simulink model "combined2"  (R2021a)
settings: Solver=VariableStepAuto  StartTime=0.0  StopTime=T_s  RelTol=1e-3
model workspace: external: MATLAB File C:\Users\abebe\Desktop\Matlab\solidworks\combined_DataFile.m (data not in the file)
values from neighbouring files (symbols this model uses):
  a_x = [0 0 0 0]    [starting_and_end_points.m]
  a_y = [10 40 30 10]    [starting_and_end_points.m]
  a_z = [30 30 30 30]    [starting_and_end_points.m]
  b_x = [0 0 0 0]    [starting_and_end_points.m]
  b_y = [40 30 10 3]    [starting_and_end_points.m]
  b_z = [30 30 30 30]    [starting_and_end_points.m]
  T = 2*max(A)    [starting_and_end_points.m]
  X = rf.*cos(PHI)    [meshing.m]
  Y = rf.*sin(PHI)    [meshing.m]
  Z = l1+(l2*sin(THETA1) + l3*sin(THETA1 + THETA2))    [meshing.m]
undefined symbols (not defined in the file or in its folder): smiData
libraries: sm_lib x20, nesl_utility x7, pid_lib x3
settings Model: Creator=Vogayer  LastModifiedBy=Vogayer

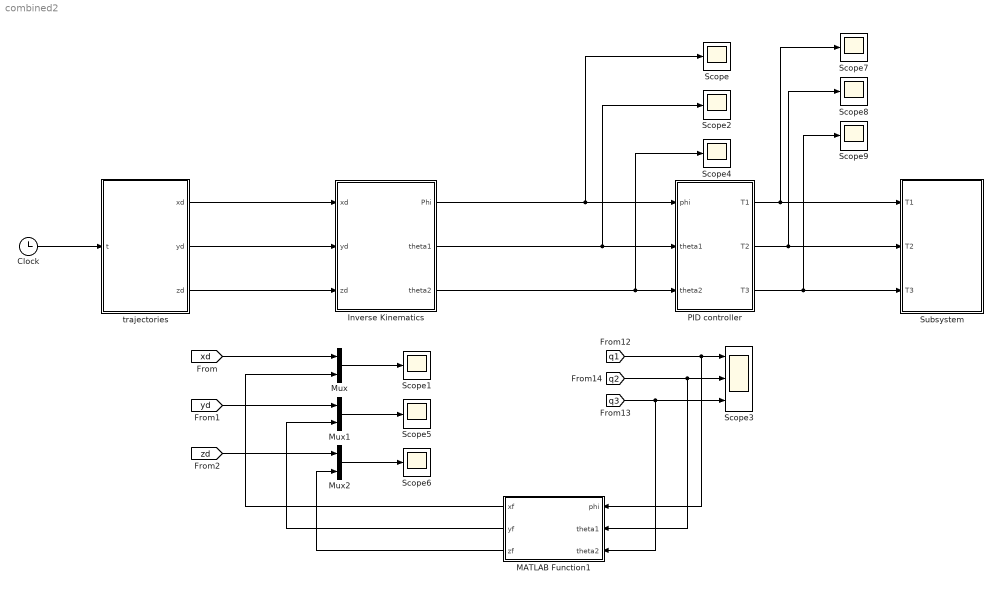
== system combined2 ==
  Clock : Clock
  Inverse Kinematics : Subsystem
  MATLAB Function1 : MATLAB Function  TreatAsAtomicUnit=on
  Mux : Mux  Inputs=2
  Mux1 : Mux  Inputs=2
  Mux2 : Mux  Inputs=2
  PID controller : Subsystem
  Scope{,1..2,4..9} (9 alike) : Scope
  Scope3 : Scope  NumInputPorts=3
  Subsystem : Subsystem
  trajectories : Subsystem
  wires:
  Inverse Kinematics/2(theta1) -> Scope2/1, PID controller/2(theta1)
  [xd] -> Mux/1
  MATLAB Function1/3(zf) -> Mux2/2
  Inverse Kinematics/3(theta2) -> Scope4/1, PID controller/3(theta2)
  MATLAB Function1/2(yf) -> Mux1/2
  [yd] -> Mux1/1
  Inverse Kinematics/1(Phi) -> Scope/1, PID controller/1(phi)
  [q2] -> MATLAB Function1/2(theta1), Scope3/2
  Mux2/1 -> Scope6/1
  [q3] -> MATLAB Function1/3(theta2), Scope3/3
  Mux/1 -> Scope1/1
  [zd] -> Mux2/1
  PID controller/1(T1) -> Subsystem/1(T1), Scope7/1
  Clock/1 -> trajectories/1(t)
  PID controller/2(T2) -> Subsystem/2(T2), Scope8/1
  Mux1/1 -> Scope5/1
  MATLAB Function1/1(xf) -> Mux/2
  [q1] -> MATLAB Function1/1(phi), Scope3/1
  PID controller/3(T3) -> Subsystem/3(T3), Scope9/1
  trajectories/1(xd) -> Inverse Kinematics/1(xd)
  trajectories/2(yd) -> Inverse Kinematics/2(yd)
  trajectories/3(zd) -> Inverse Kinematics/3(zd)

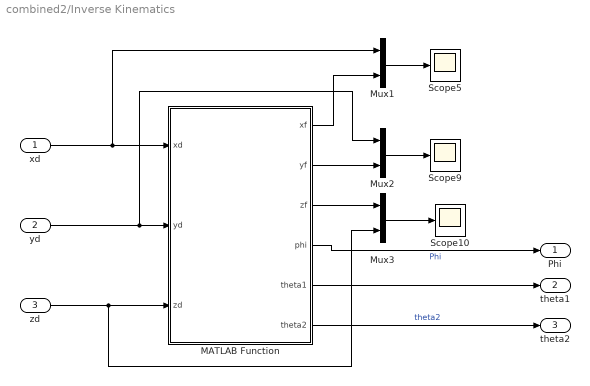
== system combined2/Inverse Kinematics ==
  xd : Inport
  yd : Inport  Port=2
  zd : Inport  Port=3
  MATLAB Function : MATLAB Function  TreatAsAtomicUnit=on
  Mux1 : Mux  Inputs=2
  Mux2 : Mux  Inputs=2
  Mux3 : Mux  Inputs=2
  Scope10 : Scope
  Scope5 : Scope
  Scope9 : Scope
  Phi : Outport
  theta1 : Outport  Port=2
  theta2 : Outport  Port=3
  wires:
  yd/1 -> MATLAB Function/2(yd), Mux2/1
  xd/1 -> MATLAB Function/1(xd), Mux1/1
  Mux2/1 -> Scope9/1
  MATLAB Function/3(zf) -> Mux3/1
  MATLAB Function/2(yf) -> Mux2/2
  Mux3/1 -> Scope10/1
  Mux1/1 -> Scope5/1
  zd/1 -> MATLAB Function/3(zd), Mux3/2
  MATLAB Function/1(xf) -> Mux1/2
  MATLAB Function/5(theta1) -> theta1/1
  MATLAB Function/4(phi) -> Phi/1  "Phi"
  MATLAB Function/6(theta2) -> theta2/1  "theta2"

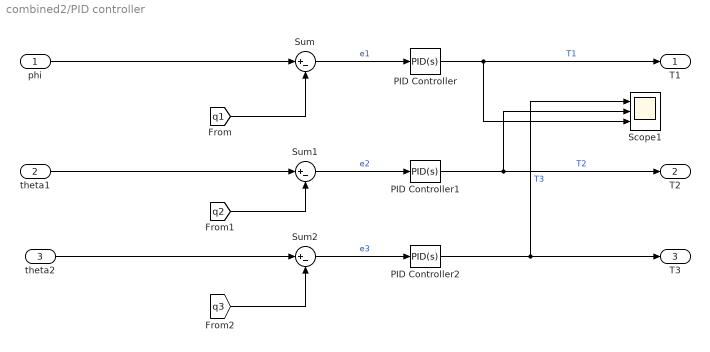
== system combined2/PID controller ==
  phi : Inport
  theta1 : Inport  Port=2
  theta2 : Inport  Port=3
  PID Controller : pid_lib/PID Controller  Controller=PID  Form=Parallel  TimeDomain=Continuous-time  UseExternalTs=off  SampleTime=-1  IntegratorMethod=Forward Euler  FilterMethod=Forward Euler  ControllerParametersSource=internal  P=2.28184982885174  I=1.06824293805434  D=1.19687109159291  UseFilter=on  N=54.5397025421619  TunerSelectOption=Transfer Function Based (PID Tuner App)  InitialConditionSource=internal  InitialConditionForIntegrator=0  InitialConditionForFilter=0  DifferentiatorICPrevScaledInput=0  ExternalReset=none  TrackingMode=off  Kt=1  LimitOutput=off  SatLimitsSource=internal  UpperSaturationLimit=inf  LowerSaturationLimit=-inf  LinearizeAsGain=on  AntiWindupMode=none  Kb=1  POutMin=[]  POutMax=[]  IOutMin=[]  IOutMax=[]  DOutMin=[]  DOutMax=[]  NOutMin=[]  NOutMax=[]  SumOutMin=[]  SumOutMax=[]  SaturationOutMin=[]  SaturationOutMax=[]  PParamMin=[]  PParamMax=[]  IParamMin=[]  IParamMax=[]  DParamMin=[]  DParamMax=[]  NParamMin=[]  NParamMax=[]  KbParamMin=[]  KbParamMax=[]  KtParamMin=[]  KtParamMax=[]  KbOutMin=[]  KbOutMax=[]  KtOutMin=[]  KtOutMax=[]  IntegratorOutMin=[]  IntegratorOutMax=[]  FilterOutMin=[]  FilterOutMax=[]  SumI1OutMin=[]  SumI1OutMax=[]  SumI2OutMin=[]  SumI2OutMax=[]  SumI3OutMin=[]  SumI3OutMax=[]  SumI4OutMin=[]  SumI4OutMax=[]  SumDOutMin=[]  SumDOutMax=[]  DifferentiatorOutMin=[]  DifferentiatorOutMax=[]  FilterDiffOutCoefMin=[]  FilterDiffOutCoefMax=[]  ReciprocalOutMin=[]  ReciprocalOutMax=[]  SumDenOutMin=[]  SumDenOutMax=[]  SumNumOutMin=[]  SumNumOutMax=[]  DivideOutMin=[]  DivideOutMax=[]  UdiffTsProdOutMin=[]  UdiffTsProdOutMax=[]  NTsProdOutMin=[]  NTsProdOutMax=[]  UintegralTsProdOutMin=[]  UintegralTsProdOutMax=[]  UngainTsProdOutMin=[]  UngainTsProdOutMax=[]  IntegratorContinuousStateAttributes=''  IntegratorStateMustResolveToSignalObject=off  IntegratorRTWStateStorageClass=Auto  FilterContinuousStateAttributes=''  FilterStateMustResolveToSignalObject=off  FilterRTWStateStorageClass=Auto  ParallelPVariant=InternalParameters  IdealPVariant=Disabled  IVariant=InternalParameters  DVariant=InternalParameters  IntegratorVariant=Continuous  SatVariant=Disabled  AWVariant=Passthrough  PCopyVariant=Disabled  TRVariant=Disabled  FdbkBlocksVariant=Forward  IdealPFdbkVariant=Disabled  SatFdbkVariant=Disabled  DerivativeFilterVariant=ContFilter  NVariant=InternalParameters  NCopyVariant=Disabled  FilterICVariant=InternalICsFilter  IntegratorICVariant=InternalICs  ExternalResetVariant=Disabled  TRSumVariant=Passthrough  SumFdbkVariant=Disabled  SumVariant=Sum_PID  TsampFilterVariant=InternalTs  TsampNgainVariant=Passthrough  TsampIntegralVariant=Passthrough  ExternalSaturationOutDataTypeStr=Inherit: Same as second input
  PID Controller1 : pid_lib/PID Controller  Controller=PID  Form=Parallel  TimeDomain=Continuous-time  UseExternalTs=off  SampleTime=-1  IntegratorMethod=Forward Euler  FilterMethod=Forward Euler  ControllerParametersSource=internal  P=66.3245976240351  I=108.858021997244  D=7.26461762494016  UseFilter=on  N=389.461376061763  TunerSelectOption=Transfer Function Based (PID Tuner App)  InitialConditionSource=internal  InitialConditionForIntegrator=0  InitialConditionForFilter=0  DifferentiatorICPrevScaledInput=0  ExternalReset=none  TrackingMode=off  Kt=1  LimitOutput=off  SatLimitsSource=internal  UpperSaturationLimit=inf  LowerSaturationLimit=-inf  LinearizeAsGain=on  AntiWindupMode=none  Kb=1  POutMin=[]  POutMax=[]  IOutMin=[]  IOutMax=[]  DOutMin=[]  DOutMax=[]  NOutMin=[]  NOutMax=[]  SumOutMin=[]  SumOutMax=[]  SaturationOutMin=[]  SaturationOutMax=[]  PParamMin=[]  PParamMax=[]  IParamMin=[]  IParamMax=[]  DParamMin=[]  DParamMax=[]  NParamMin=[]  NParamMax=[]  KbParamMin=[]  KbParamMax=[]  KtParamMin=[]  KtParamMax=[]  KbOutMin=[]  KbOutMax=[]  KtOutMin=[]  KtOutMax=[]  IntegratorOutMin=[]  IntegratorOutMax=[]  FilterOutMin=[]  FilterOutMax=[]  SumI1OutMin=[]  SumI1OutMax=[]  SumI2OutMin=[]  SumI2OutMax=[]  SumI3OutMin=[]  SumI3OutMax=[]  SumI4OutMin=[]  SumI4OutMax=[]  SumDOutMin=[]  SumDOutMax=[]  DifferentiatorOutMin=[]  DifferentiatorOutMax=[]  FilterDiffOutCoefMin=[]  FilterDiffOutCoefMax=[]  ReciprocalOutMin=[]  ReciprocalOutMax=[]  SumDenOutMin=[]  SumDenOutMax=[]  SumNumOutMin=[]  SumNumOutMax=[]  DivideOutMin=[]  DivideOutMax=[]  UdiffTsProdOutMin=[]  UdiffTsProdOutMax=[]  NTsProdOutMin=[]  NTsProdOutMax=[]  UintegralTsProdOutMin=[]  UintegralTsProdOutMax=[]  UngainTsProdOutMin=[]  UngainTsProdOutMax=[]  IntegratorContinuousStateAttributes=''  IntegratorStateMustResolveToSignalObject=off  IntegratorRTWStateStorageClass=Auto  FilterContinuousStateAttributes=''  FilterStateMustResolveToSignalObject=off  FilterRTWStateStorageClass=Auto  ParallelPVariant=InternalParameters  IdealPVariant=Disabled  IVariant=InternalParameters  DVariant=InternalParameters  IntegratorVariant=Continuous  SatVariant=Disabled  AWVariant=Passthrough  PCopyVariant=Disabled  TRVariant=Disabled  FdbkBlocksVariant=Forward  IdealPFdbkVariant=Disabled  SatFdbkVariant=Disabled  DerivativeFilterVariant=ContFilter  NVariant=InternalParameters  NCopyVariant=Disabled  FilterICVariant=InternalICsFilter  IntegratorICVariant=InternalICs  ExternalResetVariant=Disabled  TRSumVariant=Passthrough  SumFdbkVariant=Disabled  SumVariant=Sum_PID  TsampFilterVariant=InternalTs  TsampNgainVariant=Passthrough  TsampIntegralVariant=Passthrough  ExternalSaturationOutDataTypeStr=Inherit: Same as second input
  PID Controller2 : pid_lib/PID Controller  Controller=PID  Form=Parallel  TimeDomain=Continuous-time  UseExternalTs=off  SampleTime=-1  IntegratorMethod=Forward Euler  FilterMethod=Forward Euler  ControllerParametersSource=internal  P=92284.2323712411  I=28708337.0909785  D=65.6560213464691  UseFilter=on  N=51610.5658060228  TunerSelectOption=Transfer Function Based (PID Tuner App)  InitialConditionSource=internal  InitialConditionForIntegrator=0  InitialConditionForFilter=0  DifferentiatorICPrevScaledInput=0  ExternalReset=none  TrackingMode=off  Kt=1  LimitOutput=off  SatLimitsSource=internal  UpperSaturationLimit=inf  LowerSaturationLimit=-inf  LinearizeAsGain=on  AntiWindupMode=none  Kb=1  POutMin=[]  POutMax=[]  IOutMin=[]  IOutMax=[]  DOutMin=[]  DOutMax=[]  NOutMin=[]  NOutMax=[]  SumOutMin=[]  SumOutMax=[]  SaturationOutMin=[]  SaturationOutMax=[]  PParamMin=[]  PParamMax=[]  IParamMin=[]  IParamMax=[]  DParamMin=[]  DParamMax=[]  NParamMin=[]  NParamMax=[]  KbParamMin=[]  KbParamMax=[]  KtParamMin=[]  KtParamMax=[]  KbOutMin=[]  KbOutMax=[]  KtOutMin=[]  KtOutMax=[]  IntegratorOutMin=[]  IntegratorOutMax=[]  FilterOutMin=[]  FilterOutMax=[]  SumI1OutMin=[]  SumI1OutMax=[]  SumI2OutMin=[]  SumI2OutMax=[]  SumI3OutMin=[]  SumI3OutMax=[]  SumI4OutMin=[]  SumI4OutMax=[]  SumDOutMin=[]  SumDOutMax=[]  DifferentiatorOutMin=[]  DifferentiatorOutMax=[]  FilterDiffOutCoefMin=[]  FilterDiffOutCoefMax=[]  ReciprocalOutMin=[]  ReciprocalOutMax=[]  SumDenOutMin=[]  SumDenOutMax=[]  SumNumOutMin=[]  SumNumOutMax=[]  DivideOutMin=[]  DivideOutMax=[]  UdiffTsProdOutMin=[]  UdiffTsProdOutMax=[]  NTsProdOutMin=[]  NTsProdOutMax=[]  UintegralTsProdOutMin=[]  UintegralTsProdOutMax=[]  UngainTsProdOutMin=[]  UngainTsProdOutMax=[]  IntegratorContinuousStateAttributes=''  IntegratorStateMustResolveToSignalObject=off  IntegratorRTWStateStorageClass=Auto  FilterContinuousStateAttributes=''  FilterStateMustResolveToSignalObject=off  FilterRTWStateStorageClass=Auto  ParallelPVariant=InternalParameters  IdealPVariant=Disabled  IVariant=InternalParameters  DVariant=InternalParameters  IntegratorVariant=Continuous  SatVariant=Disabled  AWVariant=Passthrough  PCopyVariant=Disabled  TRVariant=Disabled  FdbkBlocksVariant=Forward  IdealPFdbkVariant=Disabled  SatFdbkVariant=Disabled  DerivativeFilterVariant=ContFilter  NVariant=InternalParameters  NCopyVariant=Disabled  FilterICVariant=InternalICsFilter  IntegratorICVariant=InternalICs  ExternalResetVariant=Disabled  TRSumVariant=Passthrough  SumFdbkVariant=Disabled  SumVariant=Sum_PID  TsampFilterVariant=InternalTs  TsampNgainVariant=Passthrough  TsampIntegralVariant=Passthrough  ExternalSaturationOutDataTypeStr=Inherit: Same as second input
  Scope1 : Scope  NumInputPorts=3
  Sum : Sum  Inputs=|+-
  Sum1 : Sum  Inputs=|+-
  Sum2 : Sum  Inputs=|+-
  T1 : Outport
  T2 : Outport  Port=2
  T3 : Outport  Port=3
  wires:
  Sum1/1 -> PID Controller1/1  "e2"
  Sum2/1 -> PID Controller2/1  "e3"
  theta2/1 -> Sum2/1
  [q3] -> Sum2/2
  [q1] -> Sum/2
  Sum/1 -> PID Controller/1  "e1"
  PID Controller2/1 -> Scope1/1, T3/1  "T3"
  phi/1 -> Sum/1
  theta1/1 -> Sum1/1
  PID Controller/1 -> T1/1, Scope1/3  "T1"
  [q2] -> Sum1/2
  PID Controller1/1 -> Scope1/2, T2/1  "T2"

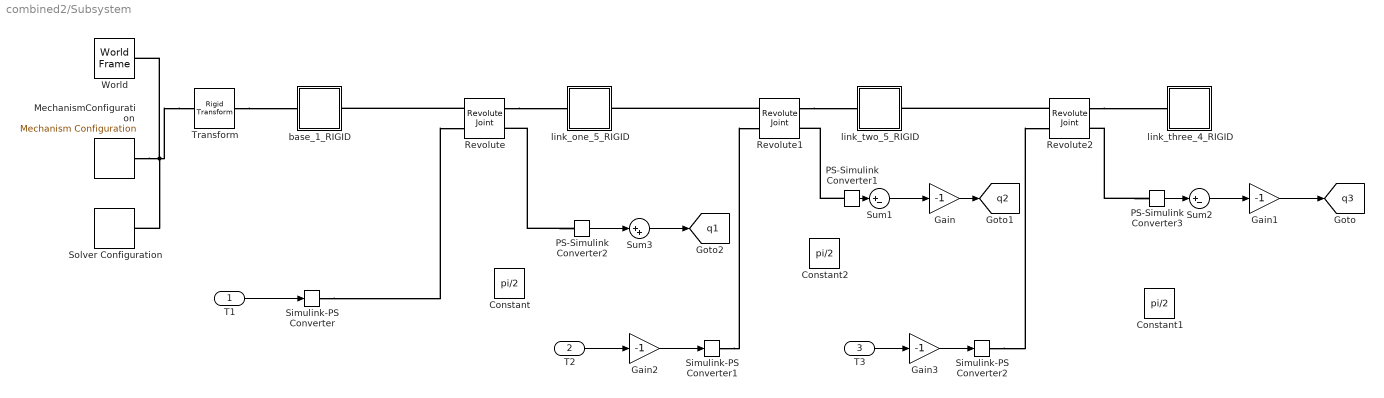
== system combined2/Subsystem ==
  T1 : Inport
  T2 : Inport  Port=2
  T3 : Inport  Port=3
  Constant : Constant  Value=pi/2
  Constant1 : Constant  Value=pi/2
  Constant2 : Constant  Value=pi/2
  Gain{,1..3} (4 alike) : Gain  Gain=-1
  MechanismConfiguration : sm_lib/Utilities/Mechanism Configuration  UniformGravity=Constant  GravityVector=[0 0 0]  GravityVectorUnits=m/s^2  GravityUnits=m/s^2  LinearizationDelta=0.001  JointModeTransitionNonlinearIterations=2
  PS-Simulink Converter1 : nesl_utility/PS-Simulink Converter  PhysicalDomain=network_engine_domain  SubClassName=ps_output  LeftPortType=input  RightPortType=output  PseudoPeriodic=off  Frequencies=[]  Unit=rad  AffineConversion=off
      settings: SourceProductBaseCode=PW,SS
  PS-Simulink Converter2 : nesl_utility/PS-Simulink Converter  PhysicalDomain=network_engine_domain  SubClassName=ps_output  LeftPortType=input  RightPortType=output  PseudoPeriodic=off  Frequencies=[]  Unit=rad  AffineConversion=off
      settings: SourceProductBaseCode=PW,SS
  PS-Simulink Converter3 : nesl_utility/PS-Simulink Converter  PhysicalDomain=network_engine_domain  SubClassName=ps_output  LeftPortType=input  RightPortType=output  PseudoPeriodic=off  Frequencies=[]  Unit=rad  AffineConversion=off
      settings: SourceProductBaseCode=PW,SS
  Revolute : sm_lib/Joints/Revolute Joint  JointMode=Normal  SenseConstraintForce=off  SenseConstraintForceX=off  SenseConstraintForceY=off  SenseConstraintForceZ=off  SenseConstraintTorque=off  SenseConstraintTorqueX=off  SenseConstraintTorqueY=off  SenseConstraintTorqueZ=off  SenseTotalForce=off  SenseTotalForceX=off  SenseTotalForceY=off  SenseTotalForceZ=off  SenseTotalTorque=off  SenseTotalTorqueX=off  SenseTotalTorqueY=off  SenseTotalTorqueZ=off  CompositeWrenchDir=FollowerOnBase  CompositeWrenchFrame=BaseFrame  EquilibriumPosition=0  EquilibriumPositionUnits=deg  SpringStiffness=0  SpringStiffnessUnits=N*m/deg  DampingCoefficient=0  DampingCoefficientUnits=N*m/(deg/s)  TorqueActuationMode=InputTorque  MotionActuationMode=ComputedMotion  SensePosition=on  SenseVelocity=off  SenseAcceleration=off  SenseTorqueForce=off  SenseLowerLimitTorqueForce=off  SenseUpperLimitTorqueForce=off  LowerLimitSpecify=off  LowerLimitBound=-90  LowerLimitBoundUnits=deg  LowerLimitStiffness=1e4  LowerLimitStiffnessUnits=N*m/deg  LowerLimitDamping=10  LowerLimitDampingUnits=N*m/(deg/s)  LowerLimitTransitionRegionWidth=0.1  LowerLimitTransitionRegionWidthUnits=deg  UpperLimitSpecify=off  UpperLimitBound=90  UpperLimitBoundUnits=deg  UpperLimitStiffness=1e4  UpperLimitStiffnessUnits=N*m/deg  UpperLimitDamping=10  UpperLimitDampingUnits=N*m/(deg/s)  UpperLimitTransitionRegionWidth=0.1  UpperLimitTransitionRegionWidthUnits=deg  PositionTargetSpecify=on  PositionTargetPriority=Low  PositionTargetValue=smiData.RevoluteJoint(1).Rz.Pos  PositionTargetValueUnits=deg  VelocityTargetSpecify=off  VelocityTargetPriority=High  VelocityTargetValue=0  VelocityTargetValueUnits=deg/s
  Revolute1 : sm_lib/Joints/Revolute Joint  JointMode=Normal  SenseConstraintForce=off  SenseConstraintForceX=off  SenseConstraintForceY=off  SenseConstraintForceZ=off  SenseConstraintTorque=off  SenseConstraintTorqueX=off  SenseConstraintTorqueY=off  SenseConstraintTorqueZ=off  SenseTotalForce=off  SenseTotalForceX=off  SenseTotalForceY=off  SenseTotalForceZ=off  SenseTotalTorque=off  SenseTotalTorqueX=off  SenseTotalTorqueY=off  SenseTotalTorqueZ=off  CompositeWrenchDir=FollowerOnBase  CompositeWrenchFrame=BaseFrame  EquilibriumPosition=0  EquilibriumPositionUnits=deg  SpringStiffness=0  SpringStiffnessUnits=N*m/deg  DampingCoefficient=0  DampingCoefficientUnits=N*m/(deg/s)  TorqueActuationMode=InputTorque  MotionActuationMode=ComputedMotion  SensePosition=on  SenseVelocity=off  SenseAcceleration=off  SenseTorqueForce=off  SenseLowerLimitTorqueForce=off  SenseUpperLimitTorqueForce=off  LowerLimitSpecify=off  LowerLimitBound=-90  LowerLimitBoundUnits=deg  LowerLimitStiffness=1e4  LowerLimitStiffnessUnits=N*m/deg  LowerLimitDamping=10  LowerLimitDampingUnits=N*m/(deg/s)  LowerLimitTransitionRegionWidth=0.1  LowerLimitTransitionRegionWidthUnits=deg  UpperLimitSpecify=off  UpperLimitBound=90  UpperLimitBoundUnits=deg  UpperLimitStiffness=1e4  UpperLimitStiffnessUnits=N*m/deg  UpperLimitDamping=10  UpperLimitDampingUnits=N*m/(deg/s)  UpperLimitTransitionRegionWidth=0.1  UpperLimitTransitionRegionWidthUnits=deg  PositionTargetSpecify=on  PositionTargetPriority=Low  PositionTargetValue=smiData.RevoluteJoint(2).Rz.Pos  PositionTargetValueUnits=deg  VelocityTargetSpecify=off  VelocityTargetPriority=High  VelocityTargetValue=0  VelocityTargetValueUnits=deg/s
  Revolute2 : sm_lib/Joints/Revolute Joint  JointMode=Normal  SenseConstraintForce=off  SenseConstraintForceX=off  SenseConstraintForceY=off  SenseConstraintForceZ=off  SenseConstraintTorque=off  SenseConstraintTorqueX=off  SenseConstraintTorqueY=off  SenseConstraintTorqueZ=off  SenseTotalForce=off  SenseTotalForceX=off  SenseTotalForceY=off  SenseTotalForceZ=off  SenseTotalTorque=off  SenseTotalTorqueX=off  SenseTotalTorqueY=off  SenseTotalTorqueZ=off  CompositeWrenchDir=FollowerOnBase  CompositeWrenchFrame=BaseFrame  EquilibriumPosition=0  EquilibriumPositionUnits=deg  SpringStiffness=0  SpringStiffnessUnits=N*m/deg  DampingCoefficient=0  DampingCoefficientUnits=N*m/(deg/s)  TorqueActuationMode=InputTorque  MotionActuationMode=ComputedMotion  SensePosition=on  SenseVelocity=off  SenseAcceleration=off  SenseTorqueForce=off  SenseLowerLimitTorqueForce=off  SenseUpperLimitTorqueForce=off  LowerLimitSpecify=off  LowerLimitBound=-90  LowerLimitBoundUnits=deg  LowerLimitStiffness=1e4  LowerLimitStiffnessUnits=N*m/deg  LowerLimitDamping=10  LowerLimitDampingUnits=N*m/(deg/s)  LowerLimitTransitionRegionWidth=0.1  LowerLimitTransitionRegionWidthUnits=deg  UpperLimitSpecify=off  UpperLimitBound=90  UpperLimitBoundUnits=deg  UpperLimitStiffness=1e4  UpperLimitStiffnessUnits=N*m/deg  UpperLimitDamping=10  UpperLimitDampingUnits=N*m/(deg/s)  UpperLimitTransitionRegionWidth=0.1  UpperLimitTransitionRegionWidthUnits=deg  PositionTargetSpecify=on  PositionTargetPriority=Low  PositionTargetValue=smiData.RevoluteJoint(3).Rz.Pos  PositionTargetValueUnits=deg  VelocityTargetSpecify=off  VelocityTargetPriority=High  VelocityTargetValue=0  VelocityTargetValueUnits=deg/s
  Simulink-PS Converter : nesl_utility/Simulink-PS Converter  PhysicalDomain=network_engine_domain  SubClassName=ps_input  LeftPortType=input  RightPortType=output  PseudoPeriodic=off  Frequencies=[]  NoiseDistribution=none  NoiseParameters=[]  Unit=N*m  AffineConversion=off  FilteringAndDerivatives=provide  SimscapeFilterOrder=1  InputFilterTimeConstant=0.001  UdotUserProvided=0
      settings: SourceProductBaseCode=PW,SS
  Simulink-PS Converter1 : nesl_utility/Simulink-PS Converter  PhysicalDomain=network_engine_domain  SubClassName=ps_input  LeftPortType=input  RightPortType=output  PseudoPeriodic=off  Frequencies=[]  NoiseDistribution=none  NoiseParameters=[]  Unit=N*m  AffineConversion=off  FilteringAndDerivatives=provide  SimscapeFilterOrder=1  InputFilterTimeConstant=0.001  UdotUserProvided=0
      settings: SourceProductBaseCode=PW,SS
  Simulink-PS Converter2 : nesl_utility/Simulink-PS Converter  PhysicalDomain=network_engine_domain  SubClassName=ps_input  LeftPortType=input  RightPortType=output  PseudoPeriodic=off  Frequencies=[]  NoiseDistribution=none  NoiseParameters=[]  Unit=N*m  AffineConversion=off  FilteringAndDerivatives=provide  SimscapeFilterOrder=1  InputFilterTimeConstant=0.001  UdotUserProvided=0
      settings: SourceProductBaseCode=PW,SS
  Solver Configuration : nesl_utility/Solver Configuration  PhysicalDomain=network_engine_domain  SubClassName=solver  LeftPortType=input  RightPortType=generic  Tones=[]  Harmonics=[]  SimulateNoise=off  Profile=off  UseLocalSampling=off  EnableSwitchedLinearOptims=on  FrequencyDomain=off  UseCCode=off  RelTol=0.001  AbsTol=1e-06  MinStep=1e-09  ToWorkspace=off  RevertToSquareIcSolve=off  NumHomotopyIterations=100  PhasorMode=off  PhasorModeNumHarmonics=1  DoDC=off  ResidualTolerance=1e-09  UseLocalSolver=off  LocalSolverChoice=NE_BACKWARD_EULER_ADVANCER  LocalSolverSampleTime=0.001  DoFixedCost=off  MaxNonlinIter=3  MaxModeIter=2  ComputeImpulses=off  ImpulseIterations=2  LinearAlgebra=auto  EquationFormulation=NE_TIME_EF  DelaysMemoryBudget=1024  AutomaticFiltering=on  FilteringTimeConstant=0.001  PartitionStorageMethod=AS_NEEDED  PartitionMemoryBudget=1024  PartitionMethod=ROBUST
      settings: SourceProductBaseCode=PW,SS
  Sum1 : Sum  Inputs=|+-
  Sum2 : Sum  Inputs=|+-
  Sum3 : Sum  Inputs=|++
  Transform : sm_lib/Frames and Transforms/Rigid Transform  TranslationMethod=Cartesian  TranslationStandardOffset=0  TranslationLengthUnit=cm  TranslationStandardAxis=+Z  TranslationCartesianOffset=smiData.RigidTransform(7).translation  TranslationROffset=0  TranslationROffsetUnits=m  TranslationZOffset=0  TranslationZOffsetUnits=m  TranslationThetaOffset=0  TranslationThetaOffsetUnits=deg  RotationMethod=ArbitraryAxis  RotationAngleUnits=rad  RotationStandardAxis=+Z  RotationAngle=smiData.RigidTransform(7).angle  RotationArbitraryAxis=smiData.RigidTransform(7).axis  FollAlignAxisA=+X  BaseAlignAxisA=+Y  FollAlignAxisB=+Y  BaseAlignAxisB=+Z  RotationSequenceAxes=FollowerAxes  RotationSequence=XYX  RotationSequenceAngles=[0 0 0]  RotationSequenceAnglesUnits=deg  RotationMatrix=[1 0 0; 0 1 0; 0 0 1]
  World : sm_lib/Frames and Transforms/World Frame
  base_1_RIGID : Subsystem
  link_one_5_RIGID : Subsystem
  link_three_4_RIGID : Subsystem
  link_two_5_RIGID : Subsystem
  tag scope: q1=global, q2=global, q3=global
  wires:
  T1/1 -> Simulink-PS Converter/1
  T3/1 -> Gain3/1
  T2/1 -> Gain2/1
  Sum3/1 -> [q1]
  Sum1/1 -> Gain/1
  PS-Simulink Converter1/1 -> Sum1/1
  PS-Simulink Converter3/1 -> Sum2/1
  PS-Simulink Converter2/1 -> Sum3/1
  Gain/1 -> [q2]
  Sum2/1 -> Gain1/1
  Gain1/1 -> [q3]
  Gain2/1 -> Simulink-PS Converter1/1
  Gain3/1 -> Simulink-PS Converter2/1
  connections:
  PS-Simulink Converter3/LConn1 -- Revolute2/RConn2
  Transform/LConn1 -- MechanismConfiguration/RConn1 -- Solver Configuration/RConn1 -- World/RConn1
  Simulink-PS Converter/RConn1 -- Revolute/LConn2
  Simulink-PS Converter2/RConn1 -- Revolute2/LConn2
  PS-Simulink Converter2/LConn1 -- Revolute/RConn2
  Revolute1/LConn1 -- link_one_5_RIGID/RConn1
  Transform/RConn1 -- base_1_RIGID/LConn1
  Revolute2/RConn1 -- link_three_4_RIGID/LConn1
  Revolute/RConn1 -- link_one_5_RIGID/LConn1
  Simulink-PS Converter1/RConn1 -- Revolute1/LConn2
  Revolute/LConn1 -- base_1_RIGID/RConn1
  PS-Simulink Converter1/LConn1 -- Revolute1/RConn2
  Revolute2/LConn1 -- link_two_5_RIGID/RConn1
  Revolute1/RConn1 -- link_two_5_RIGID/LConn1

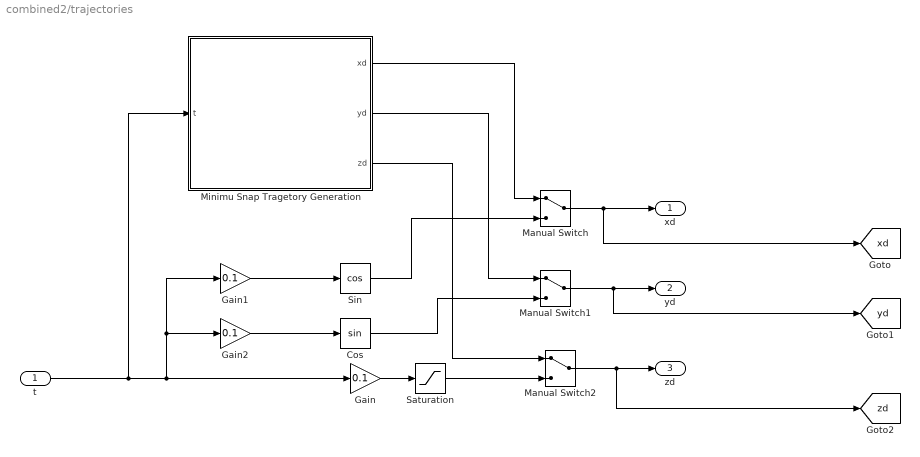
== system combined2/trajectories ==
  t : Inport
  Cos : Trigonometry
  Gain : Gain  Gain=0.1
  Gain1 : Gain  Gain=0.1
  Gain2 : Gain  Gain=0.1
  Manual Switch : ManualSwitch
  Manual Switch1 : ManualSwitch
  Manual Switch2 : ManualSwitch
  Minimu Snap Tragetory Generation : Subsystem
  Saturation : Saturate  LowerLimit=0
  Sin : Trigonometry  Operator=cos
  xd : Outport
  yd : Outport  Port=2
  zd : Outport  Port=3
  tag scope: xd=global, yd=global, zd=global
  wires:
  Cos/1 -> Manual Switch1/2
  Gain/1 -> Saturation/1
  t/1 -> Minimu Snap Tragetory Generation/1(t), Gain1/1, Gain2/1, Gain/1
  Minimu Snap Tragetory Generation/3(zd) -> Manual Switch2/1
  Minimu Snap Tragetory Generation/1(xd) -> Manual Switch/1
  Minimu Snap Tragetory Generation/2(yd) -> Manual Switch1/1
  Gain1/1 -> Sin/1
  Sin/1 -> Manual Switch/2
  Gain2/1 -> Cos/1
  Manual Switch/1 -> [xd], xd/1
  Manual Switch2/1 -> [zd], zd/1
  Manual Switch1/1 -> [yd], yd/1
  Saturation/1 -> Manual Switch2/2

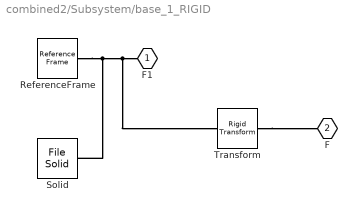
== system combined2/Subsystem/base_1_RIGID ==
  ReferenceFrame : sm_lib/Frames and Transforms/Reference Frame
  Solid : sm_lib/Body Elements/File Solid  ExtGeomFileName=base_Default_sldprt.STEP  UnitType=FromFile  ExtGeomFileUnits=m  StepReaderType=HEX  ExportConvexHullGeometry=off  InertiaType=Custom  Mass=smiData.Solid(4).mass  MassUnits=kg  CenterOfMass=smiData.Solid(4).CoM  CenterOfMassUnits=cm  MomentsOfInertia=smiData.Solid(4).MoI  MomentsOfInertiaUnits=kg*cm^2  ProductsOfInertia=smiData.Solid(4).PoI  ProductsOfInertiaUnits=kg*cm^2  BasedOnType=DensityFromFile  Density=1000  DensityUnits=kg/m^3  DoExposeReferenceFrame=on  SerializedFrames=<Frames/>  GraphicType=FromGeometry  MarkerShape=Sphere  MarkerSize=10  GraphicVisPropType=SimpleVisualProperties  GraphicDiffuseColor=smiData.Solid(4).color  GraphicSpecularColor=[0.5 0.5 0.5 1.0]  GraphicAmbientColor=[0.15 0.15 0.15 1.0]  GraphicEmissiveColor=[0.0 0.0 0.0 1.0]  GraphicShininess=75  GraphicOpacity=smiData.Solid(4).opacity
  Transform : sm_lib/Frames and Transforms/Rigid Transform  TranslationMethod=Cartesian  TranslationStandardOffset=0  TranslationLengthUnit=cm  TranslationStandardAxis=+Z  TranslationCartesianOffset=smiData.RigidTransform(1).translation  TranslationROffset=0  TranslationROffsetUnits=m  TranslationZOffset=0  TranslationZOffsetUnits=m  TranslationThetaOffset=0  TranslationThetaOffsetUnits=deg  RotationMethod=ArbitraryAxis  RotationAngleUnits=rad  RotationStandardAxis=+Z  RotationAngle=smiData.RigidTransform(1).angle  RotationArbitraryAxis=smiData.RigidTransform(1).axis  FollAlignAxisA=+X  BaseAlignAxisA=+Y  FollAlignAxisB=+Y  BaseAlignAxisB=+Z  RotationSequenceAxes=FollowerAxes  RotationSequence=XYX  RotationSequenceAngles=[0 0 0]  RotationSequenceAnglesUnits=deg  RotationMatrix=[1 0 0; 0 1 0; 0 0 1]
  F1 : PMIOPort  Side=Left
  F : PMIOPort  Port=2  Side=Right
  connections:
  Solid/RConn1 -- ReferenceFrame/RConn1 -- Transform/LConn1 -- F1/RConn1
  Transform/RConn1 -- F/RConn1

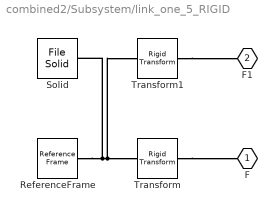
== system combined2/Subsystem/link_one_5_RIGID ==
  ReferenceFrame : sm_lib/Frames and Transforms/Reference Frame
  Solid : sm_lib/Body Elements/File Solid  ExtGeomFileName=link one_Default_sldprt.STEP  UnitType=FromFile  ExtGeomFileUnits=m  StepReaderType=HEX  ExportConvexHullGeometry=off  InertiaType=Custom  Mass=smiData.Solid(1).mass  MassUnits=kg  CenterOfMass=smiData.Solid(1).CoM  CenterOfMassUnits=cm  MomentsOfInertia=smiData.Solid(1).MoI  MomentsOfInertiaUnits=kg*cm^2  ProductsOfInertia=smiData.Solid(1).PoI  ProductsOfInertiaUnits=kg*cm^2  BasedOnType=DensityFromFile  Density=1000  DensityUnits=kg/m^3  DoExposeReferenceFrame=on  SerializedFrames=<Frames/>  GraphicType=FromGeometry  MarkerShape=Sphere  MarkerSize=10  GraphicVisPropType=SimpleVisualProperties  GraphicDiffuseColor=smiData.Solid(1).color  GraphicSpecularColor=[0.5 0.5 0.5 1.0]  GraphicAmbientColor=[0.15 0.15 0.15 1.0]  GraphicEmissiveColor=[0.0 0.0 0.0 1.0]  GraphicShininess=75  GraphicOpacity=smiData.Solid(1).opacity
  Transform : sm_lib/Frames and Transforms/Rigid Transform  TranslationMethod=Cartesian  TranslationStandardOffset=0  TranslationLengthUnit=cm  TranslationStandardAxis=+Z  TranslationCartesianOffset=smiData.RigidTransform(2).translation  TranslationROffset=0  TranslationROffsetUnits=m  TranslationZOffset=0  TranslationZOffsetUnits=m  TranslationThetaOffset=0  TranslationThetaOffsetUnits=deg  RotationMethod=ArbitraryAxis  RotationAngleUnits=rad  RotationStandardAxis=+Z  RotationAngle=smiData.RigidTransform(2).angle  RotationArbitraryAxis=smiData.RigidTransform(2).axis  FollAlignAxisA=+X  BaseAlignAxisA=+Y  FollAlignAxisB=+Y  BaseAlignAxisB=+Z  RotationSequenceAxes=FollowerAxes  RotationSequence=XYX  RotationSequenceAngles=[0 0 0]  RotationSequenceAnglesUnits=deg  RotationMatrix=[1 0 0; 0 1 0; 0 0 1]
  Transform1 : sm_lib/Frames and Transforms/Rigid Transform  TranslationMethod=Cartesian  TranslationStandardOffset=0  TranslationLengthUnit=cm  TranslationStandardAxis=+Z  TranslationCartesianOffset=smiData.RigidTransform(3).translation  TranslationROffset=0  TranslationROffsetUnits=m  TranslationZOffset=0  TranslationZOffsetUnits=m  TranslationThetaOffset=0  TranslationThetaOffsetUnits=deg  RotationMethod=ArbitraryAxis  RotationAngleUnits=rad  RotationStandardAxis=+Z  RotationAngle=smiData.RigidTransform(3).angle  RotationArbitraryAxis=smiData.RigidTransform(3).axis  FollAlignAxisA=+X  BaseAlignAxisA=+Y  FollAlignAxisB=+Y  BaseAlignAxisB=+Z  RotationSequenceAxes=FollowerAxes  RotationSequence=XYX  RotationSequenceAngles=[0 0 0]  RotationSequenceAnglesUnits=deg  RotationMatrix=[1 0 0; 0 1 0; 0 0 1]
  F : PMIOPort  Side=Left
  F1 : PMIOPort  Port=2  Side=Right
  connections:
  Solid/RConn1 -- ReferenceFrame/RConn1 -- Transform/LConn1 -- Transform1/LConn1
  Transform/RConn1 -- F/RConn1
  Transform1/RConn1 -- F1/RConn1

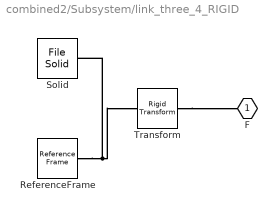
== system combined2/Subsystem/link_three_4_RIGID ==
  ReferenceFrame : sm_lib/Frames and Transforms/Reference Frame
  Solid : sm_lib/Body Elements/File Solid  ExtGeomFileName=link three_Default_sldprt.STEP  UnitType=FromFile  ExtGeomFileUnits=m  StepReaderType=HEX  ExportConvexHullGeometry=off  InertiaType=Custom  Mass=smiData.Solid(2).mass  MassUnits=kg  CenterOfMass=smiData.Solid(2).CoM  CenterOfMassUnits=cm  MomentsOfInertia=smiData.Solid(2).MoI  MomentsOfInertiaUnits=kg*cm^2  ProductsOfInertia=smiData.Solid(2).PoI  ProductsOfInertiaUnits=kg*cm^2  BasedOnType=DensityFromFile  Density=1000  DensityUnits=kg/m^3  DoExposeReferenceFrame=on  SerializedFrames=<Frames/>  GraphicType=FromGeometry  MarkerShape=Sphere  MarkerSize=10  GraphicVisPropType=SimpleVisualProperties  GraphicDiffuseColor=smiData.Solid(2).color  GraphicSpecularColor=[0.5 0.5 0.5 1.0]  GraphicAmbientColor=[0.15 0.15 0.15 1.0]  GraphicEmissiveColor=[0.0 0.0 0.0 1.0]  GraphicShininess=75  GraphicOpacity=smiData.Solid(2).opacity
  Transform : sm_lib/Frames and Transforms/Rigid Transform  TranslationMethod=Cartesian  TranslationStandardOffset=0  TranslationLengthUnit=cm  TranslationStandardAxis=+Z  TranslationCartesianOffset=smiData.RigidTransform(6).translation  TranslationROffset=0  TranslationROffsetUnits=m  TranslationZOffset=0  TranslationZOffsetUnits=m  TranslationThetaOffset=0  TranslationThetaOffsetUnits=deg  RotationMethod=ArbitraryAxis  RotationAngleUnits=rad  RotationStandardAxis=+Z  RotationAngle=smiData.RigidTransform(6).angle  RotationArbitraryAxis=smiData.RigidTransform(6).axis  FollAlignAxisA=+X  BaseAlignAxisA=+Y  FollAlignAxisB=+Y  BaseAlignAxisB=+Z  RotationSequenceAxes=FollowerAxes  RotationSequence=XYX  RotationSequenceAngles=[0 0 0]  RotationSequenceAnglesUnits=deg  RotationMatrix=[1 0 0; 0 1 0; 0 0 1]
  F : PMIOPort  Side=Left
  connections:
  Solid/RConn1 -- ReferenceFrame/RConn1 -- Transform/LConn1
  Transform/RConn1 -- F/RConn1

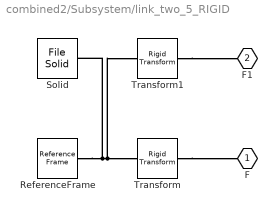
== system combined2/Subsystem/link_two_5_RIGID ==
  ReferenceFrame : sm_lib/Frames and Transforms/Reference Frame
  Solid : sm_lib/Body Elements/File Solid  ExtGeomFileName=link two_Default_sldprt.STEP  UnitType=FromFile  ExtGeomFileUnits=m  StepReaderType=HEX  ExportConvexHullGeometry=off  InertiaType=Custom  Mass=smiData.Solid(3).mass  MassUnits=kg  CenterOfMass=smiData.Solid(3).CoM  CenterOfMassUnits=cm  MomentsOfInertia=smiData.Solid(3).MoI  MomentsOfInertiaUnits=kg*cm^2  ProductsOfInertia=smiData.Solid(3).PoI  ProductsOfInertiaUnits=kg*cm^2  BasedOnType=DensityFromFile  Density=1000  DensityUnits=kg/m^3  DoExposeReferenceFrame=on  SerializedFrames=<Frames/>  GraphicType=FromGeometry  MarkerShape=Sphere  MarkerSize=10  GraphicVisPropType=SimpleVisualProperties  GraphicDiffuseColor=smiData.Solid(3).color  GraphicSpecularColor=[0.5 0.5 0.5 1.0]  GraphicAmbientColor=[0.15 0.15 0.15 1.0]  GraphicEmissiveColor=[0.0 0.0 0.0 1.0]  GraphicShininess=75  GraphicOpacity=smiData.Solid(3).opacity
  Transform : sm_lib/Frames and Transforms/Rigid Transform  TranslationMethod=Cartesian  TranslationStandardOffset=0  TranslationLengthUnit=cm  TranslationStandardAxis=+Z  TranslationCartesianOffset=smiData.RigidTransform(4).translation  TranslationROffset=0  TranslationROffsetUnits=m  TranslationZOffset=0  TranslationZOffsetUnits=m  TranslationThetaOffset=0  TranslationThetaOffsetUnits=deg  RotationMethod=ArbitraryAxis  RotationAngleUnits=rad  RotationStandardAxis=+Z  RotationAngle=smiData.RigidTransform(4).angle  RotationArbitraryAxis=smiData.RigidTransform(4).axis  FollAlignAxisA=+X  BaseAlignAxisA=+Y  FollAlignAxisB=+Y  BaseAlignAxisB=+Z  RotationSequenceAxes=FollowerAxes  RotationSequence=XYX  RotationSequenceAngles=[0 0 0]  RotationSequenceAnglesUnits=deg  RotationMatrix=[1 0 0; 0 1 0; 0 0 1]
  Transform1 : sm_lib/Frames and Transforms/Rigid Transform  TranslationMethod=Cartesian  TranslationStandardOffset=0  TranslationLengthUnit=cm  TranslationStandardAxis=+Z  TranslationCartesianOffset=smiData.RigidTransform(5).translation  TranslationROffset=0  TranslationROffsetUnits=m  TranslationZOffset=0  TranslationZOffsetUnits=m  TranslationThetaOffset=0  TranslationThetaOffsetUnits=deg  RotationMethod=ArbitraryAxis  RotationAngleUnits=rad  RotationStandardAxis=+Z  RotationAngle=smiData.RigidTransform(5).angle  RotationArbitraryAxis=smiData.RigidTransform(5).axis  FollAlignAxisA=+X  BaseAlignAxisA=+Y  FollAlignAxisB=+Y  BaseAlignAxisB=+Z  RotationSequenceAxes=FollowerAxes  RotationSequence=XYX  RotationSequenceAngles=[0 0 0]  RotationSequenceAnglesUnits=deg  RotationMatrix=[1 0 0; 0 1 0; 0 0 1]
  F : PMIOPort  Side=Left
  F1 : PMIOPort  Port=2  Side=Right
  connections:
  Solid/RConn1 -- ReferenceFrame/RConn1 -- Transform/LConn1 -- Transform1/LConn1
  Transform/RConn1 -- F/RConn1
  Transform1/RConn1 -- F1/RConn1

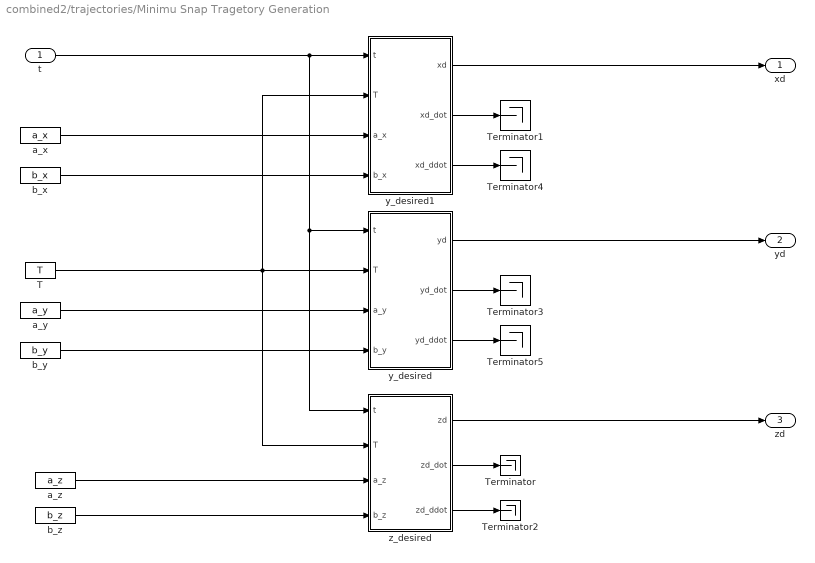
== system combined2/trajectories/Minimu Snap Tragetory Generation ==
  t : Inport
  " z_desired" : MATLAB Function  TreatAsAtomicUnit=on
  T : Constant  Value=T
  Terminator{,1..5} (6 alike) : Terminator
  a_x : Constant  Value=a_x
  a_y : Constant  Value=a_y
  a_z : Constant  Value=a_z
  b_x : Constant  Value=b_x
  b_y : Constant  Value=b_y
  b_z : Constant  Value=b_z
  y_desired : MATLAB Function  TreatAsAtomicUnit=on
  y_desired1 : MATLAB Function  TreatAsAtomicUnit=on
  xd : Outport
  yd : Outport  Port=2
  zd : Outport  Port=3
  wires:
  " z_desired"/3(zd_ddot) -> Terminator2/1
  " z_desired"/2(zd_dot) -> Terminator/1
  t/1 -> y_desired1/1(t), " z_desired"/1(t), y_desired/1(t)
  y_desired/2(yd_dot) -> Terminator3/1
  a_z/1 -> " z_desired"/3(a_z)
  T/1 -> y_desired1/2(T), " z_desired"/2(T), y_desired/2(T)
  y_desired1/1(xd) -> xd/1
  y_desired/1(yd) -> yd/1
  a_y/1 -> y_desired/3(a_y)
  b_z/1 -> " z_desired"/4(b_z)
  y_desired1/2(xd_dot) -> Terminator1/1
  " z_desired"/1(zd) -> zd/1
  b_y/1 -> y_desired/4(b_y)
  y_desired/3(yd_ddot) -> Terminator5/1
  y_desired1/3(xd_ddot) -> Terminator4/1
  a_x/1 -> y_desired1/3(a_x)
  b_x/1 -> y_desired1/4(b_x)

== matlab function combined2/Inverse Kinematics/MATLAB Function ==
  data: xd input; xf output; yd input; zd input; yf output; zf output; phi output; theta1 output; theta2 output
function [xf,yf,zf,phi,theta1,theta2] = fcn(xd,yd,zd)
l1=28;l2=40;l3=40;
phi=atan2(yd,xd);
r=sqrt(xd^2 + yd^2);
c2 = (r^2 + (zd-l1)^2 - l2^2 - l3^2)/(2*l2*l3);
s2=sqrt(1 - c2^2);
theta2=-atan2(s2,c2);
beta=-atan((l3*sin(theta2))/(l2 + l3*cos(theta2)));
gama=atan((zd-l1)/r);
theta1=gama-beta;
rf=l2*cos(theta1) + l3*cos((theta1-theta2));
zf=l1+(l2*sin(theta1) + l3*sin(theta1-theta2));
xf=rf*cos(phi);
yf=rf*sin(phi);

== matlab function combined2/MATLAB Function1 ==
  data: phi input; xf output; theta1 input; theta2 input; yf output; zf output
function [xf,yf,zf] = fcn(phi,theta1,theta2)
l1=28;l2=40;l3=40;
rf=l2*cos(theta1) + l3*cos((theta1-theta2));
zf=l1+(l2*sin(theta1) + l3*sin(theta1-theta2));
xf=rf*cos(phi);
yf=rf*sin(phi);

== matlab function combined2/trajectories/Minimu Snap Tragetory Generation/y_desired1 ==
  data: t input; T input; xd output; xd_dot output; xd_ddot output; a_x input; b_x input
function [xd,xd_dot,xd_ddot] = fcn(t,T,a_x,b_x)
if(t<=T(1,1))
T0=0;Tf=T(1,1);
a=a_x(1,1); b=b_x(1,1);
elseif(t>T(1,1)&& t<=T(2,1)+T(1,1))
T0=T(1,1);Tf=T(2,1)+T(1,1);
a=a_x(2,1); b=b_x(2,1);
elseif (t>T(2,1)+T(1,1)&& t<=T(3,1) + T(2,1)+T(1,1))
T0=T(2,1)+T(1,1);Tf=T(3,1)+ T(2,1)+T(1,1);
a=a_x(3,1); b=b_x(3,1);
else
T0=T(3,1)+ T(2,1)+T(1,1);Tf=T(4,1) + T(3,1)+ T(2,1)+T(1,1);
a=a_x(4,1); b=b_x(4,1);
end
B=[a;b;0;0;0;0;0;0];
A=[T0^6     T0^5     T0^4     T0^3    T0^2  T0^1  1;
   Tf^6     Tf^5     Tf^4     Tf^3    Tf^2  Tf^1  1;
   6*T0^5   5*T0^4   4*T0^3   3*T0^2  2*T0  1     0;
   6*Tf^5   5*Tf^4   4*Tf^3   3*Tf^2  2*Tf  1     0;
   30*T0^4  20*T0^3  12*T0^2  6*T0    2     0     0;
   30*Tf^4  20*Tf^3  12*Tf^2  6*Tf    2     0     0;
   120*T0^3  60*T0^2  24*T0   6       2     0     0;
   120*Tf^3  60*Tf^2  24*Tf   6       2     0     0];
C=A\B;
xd=C(1,1)*t^6 + C(2,1)*t^5 + C(3,1)*t^4 + C(4,1)*t^3 + C(5,1)*t^2 + C(6,1)*t + C(7,1);
xd_dot=6*C(1,1)*t^5 + 5*C(2,1)*t^4  + 4*C(3,1)*t^3 + 3*C(4,1)*t^2 + 2*C(5,1)*t + C(6,1);
xd_ddot=30*C(1,1)*t^4 + 20*C(2,1)*t^3  + 12*C(3,1)*t^2 + 6*C(4,1)*t + 2*C(5,1);

== matlab function combined2/trajectories/Minimu Snap Tragetory Generation/y_desired ==
  data: t input; T input; yd output; yd_dot output; yd_ddot output; a_y input; b_y input
function [yd,yd_dot,yd_ddot] = fcn(t,T,a_y,b_y)
if(t<=T(1,1))
T0=0;Tf=T(1,1);
a=a_y(1,1); b=b_y(1,1);
elseif(t>T(1,1)&& t<=T(2,1)+T(1,1))
T0=T(1,1);Tf=T(2,1)+T(1,1);
a=a_y(2,1); b=b_y(2,1);
elseif (t>T(2,1)+T(1,1)&& t<=T(3,1) + T(2,1)+T(1,1))
T0=T(2,1)+T(1,1);Tf=T(3,1)+ T(2,1)+T(1,1);
a=a_y(3,1); b=b_y(3,1);
else
T0=T(3,1)+ T(2,1)+T(1,1);Tf=T(4,1) + T(3,1)+ T(2,1)+T(1,1);
a=a_y(4,1); b=b_y(4,1);
end
B=[a;b;0;0;0;0;0;0];
A=[T0^6     T0^5     T0^4     T0^3    T0^2  T0^1  1;
   Tf^6     Tf^5     Tf^4     Tf^3    Tf^2  Tf^1  1;
   6*T0^5   5*T0^4   4*T0^3   3*T0^2  2*T0  1     0;
   6*Tf^5   5*Tf^4   4*Tf^3   3*Tf^2  2*Tf  1     0;
   30*T0^4  20*T0^3  12*T0^2  6*T0    2     0     0;
   30*Tf^4  20*Tf^3  12*Tf^2  6*Tf    2     0     0;
   120*T0^3  60*T0^2  24*T0   6       2     0     0;
   120*Tf^3  60*Tf^2  24*Tf   6       2     0     0];
C=A\B;
yd=C(1,1)*t^6 + C(2,1)*t^5 + C(3,1)*t^4 + C(4,1)*t^3 + C(5,1)*t^2 + C(6,1)*t + C(7,1);
yd_dot=6*C(1,1)*t^5 + 5*C(2,1)*t^4  + 4*C(3,1)*t^3 + 3*C(4,1)*t^2 + 2*C(5,1)*t + C(6,1);
yd_ddot=30*C(1,1)*t^4 + 20*C(2,1)*t^3  + 12*C(3,1)*t^2 + 6*C(4,1)*t + 2*C(5,1);

== matlab function combined2/trajectories/Minimu Snap Tragetory Generation/ z_desired ==
  data: t input; T input; zd output; zd_dot output; zd_ddot output; a_z input; b_z input
function [zd,zd_dot,zd_ddot] = fcn(t,T,a_z,b_z)
if(t<=T(1,1))
T0=0;Tf=T(1,1);
a=a_z(1,1); b=b_z(1,1);
elseif(t>T(1,1)&& t<=T(2,1)+T(1,1))
T0=T(1,1);Tf=T(2,1)+T(1,1);
a=a_z(2,1); b=b_z(2,1);
elseif (t>T(2,1)+T(1,1)&& t<=T(3,1) + T(2,1)+T(1,1))
T0=T(2,1)+T(1,1);Tf=T(3,1)+ T(2,1)+T(1,1);
a=a_z(3,1); b=b_z(3,1);
else
T0=T(3,1)+ T(2,1)+T(1,1);Tf=T(4,1) + T(3,1)+ T(2,1)+T(1,1);
a=a_z(4,1); b=b_z(4,1);
end
B=[a;b;0;0;0;0;0;0];
A=[T0^6     T0^5     T0^4     T0^3    T0^2  T0^1  1;
   Tf^6     Tf^5     Tf^4     Tf^3    Tf^2  Tf^1  1;
   6*T0^5   5*T0^4   4*T0^3   3*T0^2  2*T0  1     0;
   6*Tf^5   5*Tf^4   4*Tf^3   3*Tf^2  2*Tf  1     0;
   30*T0^4  20*T0^3  12*T0^2  6*T0    2     0     0;
   30*Tf^4  20*Tf^3  12*Tf^2  6*Tf    2     0     0;
   120*T0^3  60*T0^2  24*T0   6       2     0     0;
   120*Tf^3  60*Tf^2  24*Tf   6       2     0     0];
C=A\B;
zd=C(1,1)*t^6 + C(2,1)*t^5 + C(3,1)*t^4 + C(4,1)*t^3 + C(5,1)*t^2 + C(6,1)*t + C(7,1);
zd_dot=6*C(1,1)*t^5 + 5*C(2,1)*t^4  + 4*C(3,1)*t^3 + 3*C(4,1)*t^2 + 2*C(5,1)*t + C(6,1);
zd_ddot=30*C(1,1)*t^4 + 20*C(2,1)*t^3  + 12*C(3,1)*t^2 + 6*C(4,1)*t + 2*C(5,1);
